simulink library "Tower_org"  (Simulink 10.0)
settings: Solver=ode45  StartTime=0.0  StopTime=10.0  RelTol=1e-3  EnableMultiTasking=on
undefined symbols (not defined in the file): WT_Params, X, Y, Z
libraries: sm_lib x5
Description:
  | Copyright 2009-2017 The MathWorks, Inc. MathWorks, Inc.
settings Model: Creator=smiller  LastModifiedBy=annonymous

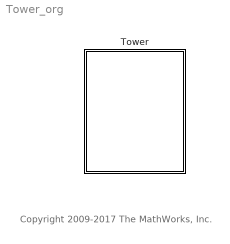
== system Tower_org ==
  note: Copyright 2009-2017 The MathWorks, Inc.
  Tower : Subsystem
      mask Display:
      | image(imread('Tower_IMAGE.jpg'));
      | port_label('RConn',1,'Env');
      | port_label('RConn',2,'GrVa');
      | port_label('RConn',3,'GrVb');
      | port_label('RConn',4,'GrVc');
      | port_label('LConn',1,'N');
      | port_label('LConn',2,'GrVa');
      | port_label('LConn',3,'GrVb');
      | port_label('LConn',4,'GrVc');

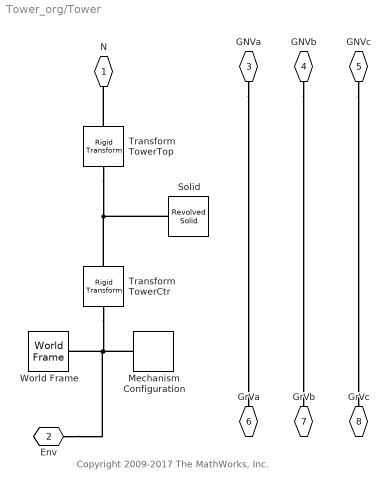
== system Tower_org/Tower ==
  note: Copyright 2009-2017 The MathWorks, Inc.
  Mechanism Configuration : sm_lib/Utilities/Mechanism Configuration  UniformGravity=Constant  GravityVector=[0 0 -9.81]*0  GravityUnits=m/s^2  LinearizationDelta=0.001
  Solid : sm_lib/Body Elements/Revolved Solid  GraphicAmbientColor=[0.15 0.15 0.15 1.0]  BasedOnType=Density  CenterOfMass=[0 0 0]  CenterOfMassUnits=m  GraphicDiffuseColor=[0.8 0.8 0.8]  Density=1000  DensityUnits=kg/(m^3)  DoExposeReferenceFrame=on  GraphicEmissiveColor=[0.0 0.0 0.0 1.0]  ExportEntireGeometry=off  SerializedFrames=<Frames/>  MarkerShape=Sphere  MarkerSize=10  GraphicType=FromGeometry  InertiaType=CalculateFromGeometry  Mass=1  MassUnits=kg  MomentsOfInertia=[1 1 1]  MomentsOfInertiaUnits=kg*m^2  GraphicOpacity=1.0  ProductsOfInertia=[0 0 0]  ProductsOfInertiaUnits=kg*m^2  RevolutionCrossSection=[0 -WT_Params.Tower.height/2;WT_Params.Tower.base_radius -WT_Params.Tower.height/2;WT_Params.Tower.top_radius WT_Params.Tower.height/2;0 WT_Params.Tower.height/2]  RevolutionCrossSectionUnits=m  RevolutionAngle=180  RevolutionAngleUnits=deg  RevolutionExtent=Full  GraphicShininess=75  GraphicSpecularColor=[0.5 0.5 0.5 1.0]  GraphicVisPropType=SimpleVisualProperties
      settings: SourceProductName=Simscape Multibody
  Transform TowerCtr : sm_lib/Frames and Transforms/Rigid Transform  TranslationMethod=StandardAxis  TranslationStandardOffset=WT_Params.Tower.height/2  TranslationLengthUnit=m  TranslationStandardAxis=+Z  TranslationCartesianOffset=[0 0 0]  TranslationROffset=0  TranslationROffsetUnits=m  TranslationZOffset=0  TranslationZOffsetUnits=m  TranslationThetaOffset=0  TranslationThetaOffsetUnits=deg  RotationMethod=None  RotationAngleUnits=deg  RotationStandardAxis=+Z  RotationAngle=0  RotationArbitraryAxis=[0 0 1]  FollAlignAxisA=+X  BaseAlignAxisA=+Y  FollAlignAxisB=+Y  BaseAlignAxisB=+Z  RotationSequenceAxes=FollowerAxes  RotationSequence=XYX  RotationSequenceAngles=[0 0 0]  RotationSequenceAnglesUnits=deg  RotationMatrix=[1 0 0; 0 1 0; 0 0 1]
  Transform TowerTop : sm_lib/Frames and Transforms/Rigid Transform  TranslationMethod=StandardAxis  TranslationStandardOffset=WT_Params.Tower.height/2  TranslationLengthUnit=m  TranslationStandardAxis=+Z  TranslationCartesianOffset=[0 0 0]  TranslationROffset=0  TranslationROffsetUnits=m  TranslationZOffset=0  TranslationZOffsetUnits=m  TranslationThetaOffset=0  TranslationThetaOffsetUnits=deg  RotationMethod=None  RotationAngleUnits=deg  RotationStandardAxis=+Z  RotationAngle=0  RotationArbitraryAxis=[0 0 1]  FollAlignAxisA=+X  BaseAlignAxisA=+Y  FollAlignAxisB=+Y  BaseAlignAxisB=+Z  RotationSequenceAxes=FollowerAxes  RotationSequence=XYX  RotationSequenceAngles=[0 0 0]  RotationSequenceAnglesUnits=deg  RotationMatrix=[1 0 0; 0 1 0; 0 0 1]
  World Frame : sm_lib/Frames and Transforms/World Frame
  N : PMIOPort  Side=Left
  Env : PMIOPort  Port=2  Side=Right
  GNVa : PMIOPort  Tag=PMCPort  Port=3  Side=Left
  GNVb : PMIOPort  Tag=PMCPort  Port=4  Side=Left
  GNVc : PMIOPort  Tag=PMCPort  Port=5  Side=Left
  GrVa : PMIOPort  Tag=PMCPort  Port=6  Side=Right
  GrVb : PMIOPort  Tag=PMCPort  Port=7  Side=Right
  GrVc : PMIOPort  Tag=PMCPort  Port=8  Side=Right
  connections:
  Solid/RConn1 -- Transform TowerTop/LConn1 -- Transform TowerCtr/RConn1
  Transform TowerTop/RConn1 -- N/RConn1
  Transform TowerCtr/LConn1 -- Env/RConn1 -- World Frame/RConn1 -- Mechanism Configuration/RConn1
  GNVc/RConn1 -- GrVc/RConn1
  GNVb/RConn1 -- GrVb/RConn1
  GNVa/RConn1 -- GrVa/RConn1
